simulink model "platoon"  (R2016a)
settings: Solver=VariableStepAuto  StartTime=0.0  StopTime=8  RelTol=1e-3
StartFcn:
  | global mdl;
  | mdl = run_setup;
settings Model: Creator=swsmth  LastModifiedBy=swsmth
settings GRTTargetCC: GeneratePreprocessorConditionals=Use local settings

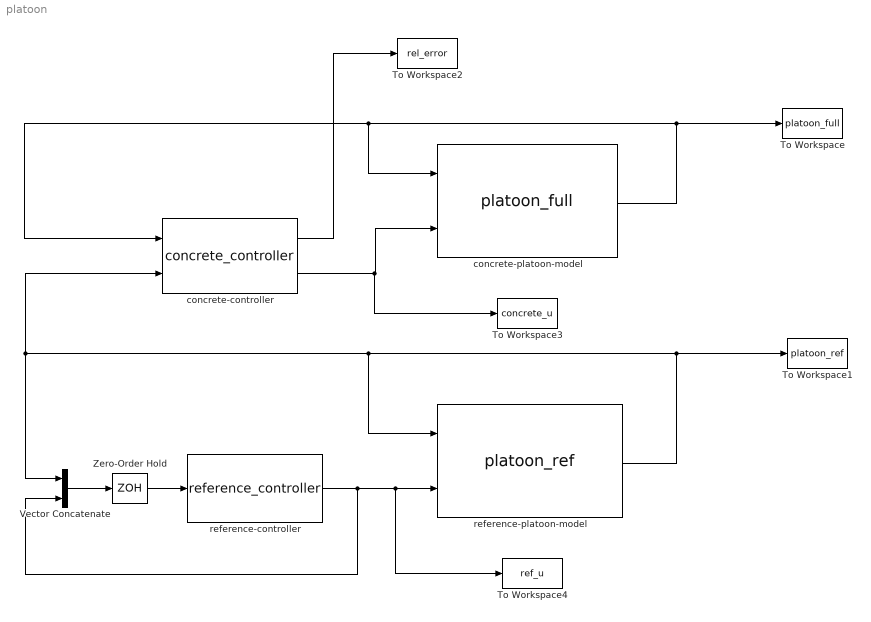
== system platoon ==
  To Workspace : ToWorkspace  VariableName=platoon_full  SampleTime=-1
  To Workspace1 : ToWorkspace  VariableName=platoon_ref  SampleTime=-1
  To Workspace2 : ToWorkspace  VariableName=rel_error  SampleTime=-1
  To Workspace3 : ToWorkspace  VariableName=concrete_u  SampleTime=-1
  To Workspace4 : ToWorkspace  VariableName=ref_u  SampleTime=-1
  Vector Concatenate : Concatenate
  Zero-Order Hold : ZeroOrderHold  SampleTime=.01
  concrete-controller : M-S-Function  FunctionName=concrete_controller
  concrete-platoon-model : M-S-Function  FunctionName=platoon_full
  reference-controller : M-S-Function  FunctionName=reference_controller
  reference-platoon-model : M-S-Function  FunctionName=platoon_ref
  wires:
  concrete-platoon-model/1 -> concrete-controller/1, concrete-platoon-model/1, To Workspace/1
  reference-platoon-model/1 -> To Workspace1/1, reference-platoon-model/1, Vector Concatenate/1, concrete-controller/2
  Zero-Order Hold/1 -> reference-controller/1
  concrete-controller/1 -> To Workspace2/1
  concrete-controller/2 -> To Workspace3/1, concrete-platoon-model/2
  reference-controller/1 -> Vector Concatenate/2, To Workspace4/1, reference-platoon-model/2
  Vector Concatenate/1 -> Zero-Order Hold/1
